simulink model "manitius_ex1_simu"  (R2023a)
settings: Solver=VariableStepAuto  StartTime=0.0  StopTime=Tsim  RelTol=1e-3
values from neighbouring files (symbols this model uses):
  A = block.DialogPrm(2).Data    [IntW.m]    (also in manitius_ex1_code.m = [0 0; 1 1])
  A1z = dssP1.A    [manitius_ex1_code.m]    (also in manitius_ex2_code.m)
  A2z = dssP2.A    [manitius_ex1_code.m]
  B1 = [1; 0]    [manitius_ex1_code.m]
  B1z = dssP1.B    [manitius_ex1_code.m]    (also in manitius_ex2_code.m)
  B2z = dssP2.B    [manitius_ex1_code.m]
  C1z = dssP1.C    [manitius_ex1_code.m]    (also in manitius_ex2_code.m)
  C2z = dssP2.C    [manitius_ex1_code.m]
  F = double(subs(F))    [manitius_ex1_code.m]
  h = 2    [manitius_ex1_code.m]    (also in manitius_ex2_code.m)
  N = block.DialogPrm(5).Data    [IntW.m]    (also in manitius_ex1_code.m = 1000; manitius_ex2_code.m = 2000)
undefined symbols (not defined in the file or in its folder): Ad1, Ad2, Bd1, Bd2, Cd1, Cd2, Dd1, Dd2, KSum1, KSum2, Q1, Q2, tal1, tal2
libraries: cstblocks x1
settings Model: Creator=Vasco  LastModifiedBy=Vasco
settings DataIOCC: ReturnWorkspaceOutputs=off

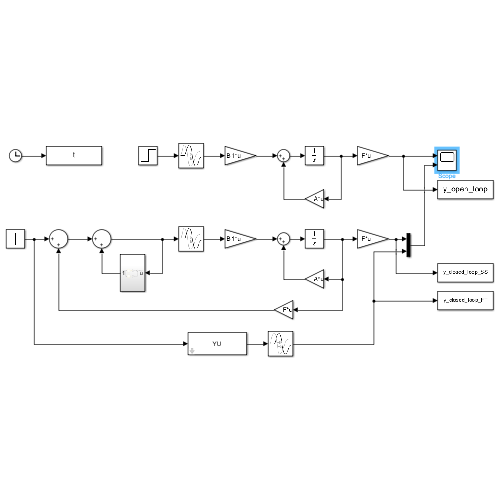
[thumbnail: Simulink's stored preview of the top-level diagram]
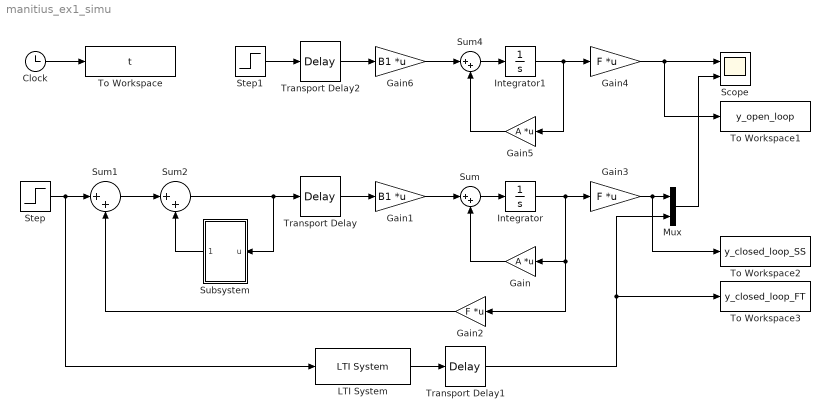
== system manitius_ex1_simu ==
  Clock : Clock
  Gain : Gain  Gain=A  Multiplication=Matrix(K*u)
  Gain1 : Gain  Gain=B1  Multiplication=Matrix(K*u)
  Gain2 : Gain  Gain=F  Multiplication=Matrix(K*u)
  Gain3 : Gain  Gain=F  Multiplication=Matrix(K*u)
  Gain4 : Gain  Gain=F  Multiplication=Matrix(K*u)
  Gain5 : Gain  Gain=A  Multiplication=Matrix(K*u)
  Gain6 : Gain  Gain=B1  Multiplication=Matrix(K*u)
  Integrator : Integrator
  Integrator1 : Integrator
  LTI System : cstblocks/LTI System  sys=YU  IC=[]
  Mux : Mux  Inputs=2
  Scope : Scope  NumInputPorts=2
  Step : Step  Time=0  SampleTime=0
  Step1 : Step  Time=0  SampleTime=0
  Subsystem : Subsystem
  Sum{,1..2,4} (4 alike) : Sum  Inputs=|++
  To Workspace : ToWorkspace  VariableName=t  SampleTime=-1
  To Workspace1 : ToWorkspace  VariableName=y_open_loop  SampleTime=-1
  To Workspace2 : ToWorkspace  VariableName=y_closed_loop_SS  SampleTime=-1
  To Workspace3 : ToWorkspace  VariableName=y_closed_loop_FT  SampleTime=-1
  Transport Delay : TransportDelay  DelayTime=h
  Transport Delay1 : TransportDelay  DelayTime=h
  Transport Delay2 : TransportDelay  DelayTime=h
  wires:
  Sum/1 -> Integrator/1
  Gain/1 -> Sum/2
  Gain2/1 -> Sum1/2
  Step/1 -> Sum1/1, LTI System/1
  Integrator/1 -> Gain2/1, Gain/1, Gain3/1
  LTI System/1 -> Transport Delay1/1
  Transport Delay1/1 -> Mux/2, To Workspace3/1
  Transport Delay/1 -> Gain1/1
  Gain1/1 -> Sum/1
  Gain3/1 -> To Workspace2/1, Mux/1
  Sum2/1 -> Subsystem/1(u), Transport Delay/1
  Sum1/1 -> Sum2/1
  Subsystem/1(Out1) -> Sum2/2
  Step1/1 -> Transport Delay2/1
  Clock/1 -> To Workspace/1
  Transport Delay2/1 -> Gain6/1
  Integrator1/1 -> Gain4/1, Gain5/1
  Gain6/1 -> Sum4/1
  Sum4/1 -> Integrator1/1
  Gain5/1 -> Sum4/2
  Mux/1 -> Scope/2
  Gain4/1 -> To Workspace1/1, Scope/1

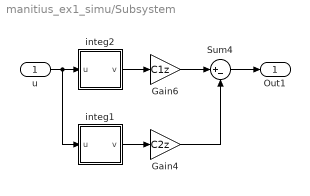
== system manitius_ex1_simu/Subsystem ==
  u : Inport
  Gain4 : Gain  Gain=C2z
  Gain6 : Gain  Gain=C1z
  Sum4 : Sum  Inputs=|+-
  integ1 : Subsystem
  integ2 : Subsystem
  Out1 : Outport
  wires:
  Gain4/1 -> Sum4/2
  u/1 -> integ1/1(u), integ2/1(u)
  integ2/1(v) -> Gain6/1
  Sum4/1 -> Out1/1
  Gain6/1 -> Sum4/1
  integ1/1(v) -> Gain4/1

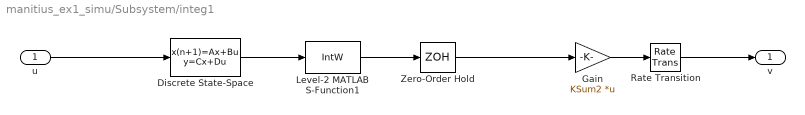
== system manitius_ex1_simu/Subsystem/integ1 ==
  u : Inport
  Discrete State-Space : DiscreteStateSpace  A=Ad2  B=Bd2  C=Cd2  D=Dd2  SampleTime=tal2
  Gain : Gain  Gain=KSum2  Multiplication=Matrix(K*u)
  Level-2 MATLAB S-Function1 : M-S-Function  FunctionName=IntW  Parameters=tal2,A2z,B2z,Q2,N
  Rate Transition : RateTransition
  Zero-Order Hold : ZeroOrderHold  SampleTime=tal2
  v : Outport  VectorParamsAs1DForOutWhenUnconnected=off
  wires:
  Rate Transition/1 -> v/1
  u/1 -> Discrete State-Space/1
  Gain/1 -> Rate Transition/1
  Zero-Order Hold/1 -> Gain/1
  Discrete State-Space/1 -> Level-2 MATLAB S-Function1/1
  Level-2 MATLAB S-Function1/1 -> Zero-Order Hold/1

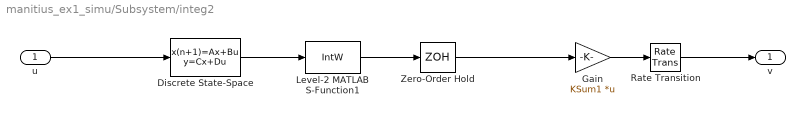
== system manitius_ex1_simu/Subsystem/integ2 ==
  u : Inport
  Discrete State-Space : DiscreteStateSpace  A=Ad1  B=Bd1  C=Cd1  D=Dd1  SampleTime=tal1
  Gain : Gain  Gain=KSum1  Multiplication=Matrix(K*u)
  Level-2 MATLAB S-Function1 : M-S-Function  FunctionName=IntW  Parameters=tal1,A1z,B1z,Q1,N
  Rate Transition : RateTransition
  Zero-Order Hold : ZeroOrderHold  SampleTime=tal1
  v : Outport  VectorParamsAs1DForOutWhenUnconnected=off
  wires:
  Rate Transition/1 -> v/1
  u/1 -> Discrete State-Space/1
  Gain/1 -> Rate Transition/1
  Zero-Order Hold/1 -> Gain/1
  Discrete State-Space/1 -> Level-2 MATLAB S-Function1/1
  Level-2 MATLAB S-Function1/1 -> Zero-Order Hold/1
